simulink model "complete_model"  (R2023b)
settings: Solver=ode5  StartTime=0.0  StopTime=1000  RelTol=1e-3
values from neighbouring files (symbols this model uses):
  a = 6851.22197053    [IGRF13_2020.mat]    (also in complete_model.m; complete_model_main.m; loop_model.m; orbit_plot_report.m)
  alpha1 = 0.4    [IGRF13_2020.mat]    (also in complete_model.m = 0.05; complete_model_main.m; loop_model.m)
  alpha2 = 0.1    [IGRF13_2020.mat]    (also in complete_model.m = 0.15; complete_model_main.m; loop_model.m)
  alpha3 = 0.5    [IGRF13_2020.mat]    (also in complete_model.m = 0.8; complete_model_main.m; loop_model.m)
  e = 0.00183012221618    [IGRF13_2020.mat]    (also in complete_model.m; complete_model_main.m; loop_model.m; orbit_plot_report.m)
  FOV_earth = 0.575958653158    [IGRF13_2020.mat]    (also in complete_model.m = deg2rad(33); complete_model_main.m = deg2rad(33); loop_model.m = deg2rad(33))
  FOV_sun = deg2rad(85)    [complete_model_main.m]
  freq_earth = 30    [IGRF13_2020.mat]    (also in complete_model.m; complete_model_main.m = 5; loop_model.m)
  freq_mag = 30    [IGRF13_2020.mat]    (also in complete_model.m; complete_model_main.m = 5; loop_model.m)
  freq_sun = 30    [IGRF13_2020.mat]    (also in complete_model.m; complete_model_main.m = 5; loop_model.m)
  H0 = 2.98059244128e-05    [IGRF13_2020.mat]    (also in complete_model.m = sqrt(g01^2+g11^2+h11^2)*1e-9; complete_model_main.m = sqrt(g01^2+g11^2+h11^2)*1e-9; loop_model.m = sqrt(g01^2+g11^2+h11^2)*1e-9)
  I = diag([I1 I2 I3])    [complete_model_main.m]
  Iinv = I\eye(3)    [complete_model_main.m]
  incl = 0.200712863979    [IGRF13_2020.mat]    (also in complete_model.m = deg2rad(11.5); complete_model_main.m = deg2rad(11.5); loop_model.m = deg2rad(11.5))
  jb = [0.01 0.05 0.01]    [IGRF13_2020.mat]    (also in complete_model.m = [0.01; 0.05; 0.01]; complete_model_main.m = [0.01; 0.05; 0.01]; loop_model.m = [0.01; 0.05; 0.01])
  k_gain = 0.0363323388759    [IGRF13_2020.mat]    (also in complete_model.m = (4*pi/T) * (1 + sin(chsi)) * I1_retr; complete_model_main.m = (4*pi/T) * (1 + sin(chsi)) * min([I1, I2, I3]); loop_model.m = (4*pi/T) * (1 + sin(chsi)) * I1_retr)
  max_dip = 15    [IGRF13_2020.mat]    (also in complete_model.m; complete_model_main.m = 150; loop_model.m)
  mu = 398600.433    [IGRF13_2020.mat]    (also in complete_model.m = astroConstants(13); complete_model_main.m = astroConstants(13); loop_model.m = astroConstants(13); orbit_plot_report.m = astroConstants(13))
  n = 0.00111331183439    [IGRF13_2020.mat]    (also in complete_model.m = sqrt(mu/a^3); complete_model_main.m = sqrt(mu/a^3); loop_model.m = sqrt(mu/a^3); orbit_plot_report.m = sqrt(mu/a^3))
  omega0 = [0.06 0.06 0.06]    [IGRF13_2020.mat]    (also in complete_model.m = -0.06 + 0.12 * rand(3,1); complete_model_main.m = [0.01; 0.01; 0.01]*6; init_cond.mat = [-0.0472016675783 0.0554277697026 -0.0594438931039]; loop_model.m = 0.06 * ones(3,1))
  omegaE = 7.27220521664e-05    [IGRF13_2020.mat]    (also in complete_model.m = deg2rad(15)/3600; complete_model_main.m = deg2rad(15)/3600; loop_model.m = deg2rad(15)/3600)
  rs = [-16878165.0145 -134206589.72 -58177126.6728]    [IGRF13_2020.mat]    (also in complete_model.m = -rr; complete_model_main.m = -rr; loop_model.m = -rr; orbit_plot_report.m = -rr)
  Rt = 6371.01    [IGRF13_2020.mat]    (also in Terra_3D.m = 6378.1363; complete_model.m = astroConstants(23); complete_model_main.m = astroConstants(23); loop_model.m = astroConstants(23))
  s0 = [6.01405730572 3.04970514452 5.02831048374]    [IGRF13_2020.mat]    (also in buonnatale.mat = [2.59731710564 0.831637671153 -2.52872821404]; complete_model.m = 2*pi*rand(3,1); complete_model_main.m = -pi + 2 * pi * rand(3,1); init_cond.mat = [4.86890604626 5.13526758752 5.45816980916])
  tol = 0.2    [IGRF13_2020.mat]    (also in complete_model.m; complete_model_main.m; loop_model.m)
undefined symbols (not defined in the file or in its folder): magnitude
libraries: matrix_library x8, vrlib x8, simulink x7, sharedutil x2, dspmathops x2, dspfactors x1, cstblocks x1
(part 2 of 2)

== system complete_model/Kinematics/Kinematics 313/s_312 - A/R2 ==
  x : Inport
  Constant : Constant  Value=[0; 1; 0]
  Constant1 : Constant  Value=0
  Cos : Trigonometry  Operator=cos
  Gain : Gain  Gain=-1
  Matrix Concatenate : Concatenate  NumInputs=3  Mode=Multidimensional array  ConcatenateDimension=2
  Sin : Trigonometry
  Vector Concatenate : Concatenate  NumInputs=3
  Vector Concatenate1 : Concatenate  NumInputs=3
  R2 : Outport
  wires:
  Vector Concatenate/1 -> Matrix Concatenate/1
  x/1 -> Sin/1, Cos/1
  Matrix Concatenate/1 -> R2/1
  Constant/1 -> Matrix Concatenate/2
  Vector Concatenate1/1 -> Matrix Concatenate/3
  Constant1/1 -> Vector Concatenate/2, Vector Concatenate1/2
  Cos/1 -> Vector Concatenate1/3, Vector Concatenate/1
  Sin/1 -> Gain/1, Vector Concatenate/3
  Gain/1 -> Vector Concatenate1/1

== system complete_model/Kinematics/Kinematics 313/s_312 - A/R3 ==
  x : Inport
  Constant : Constant  Value=[0; 0; 1]
  Constant1 : Constant  Value=0
  Cos : Trigonometry  Operator=cos
  Gain : Gain  Gain=-1
  Matrix Concatenate : Concatenate  NumInputs=3  Mode=Multidimensional array  ConcatenateDimension=2
  Sin : Trigonometry
  Vector Concatenate : Concatenate  NumInputs=3
  Vector Concatenate1 : Concatenate  NumInputs=3
  R3 : Outport
  wires:
  Vector Concatenate/1 -> Matrix Concatenate/1
  Sin/1 -> Vector Concatenate1/1, Gain/1
  Cos/1 -> Vector Concatenate1/2, Vector Concatenate/1
  Constant/1 -> Matrix Concatenate/3
  Gain/1 -> Vector Concatenate/2
  Vector Concatenate1/1 -> Matrix Concatenate/2
  x/1 -> Sin/1, Cos/1
  Constant1/1 -> Vector Concatenate/3, Vector Concatenate1/3
  Matrix Concatenate/1 -> R3/1

== system complete_model/Kinematics/Kinematics 313/s_313 - A/R1 ==
  x : Inport
  Constant : Constant  Value=[1; 0; 0]
  Constant1 : Constant  Value=0
  Cos : Trigonometry  Operator=cos
  Gain : Gain  Gain=-1
  Matrix Concatenate : Concatenate  NumInputs=3  Mode=Multidimensional array  ConcatenateDimension=2
  Sin : Trigonometry
  Vector Concatenate : Concatenate  NumInputs=3
  Vector Concatenate1 : Concatenate  NumInputs=3
  R1 : Outport
  wires:
  Sin/1 -> Gain/1, Vector Concatenate/2
  Gain/1 -> Vector Concatenate1/3
  Cos/1 -> Vector Concatenate1/2, Vector Concatenate/3
  Constant1/1 -> Vector Concatenate1/1, Vector Concatenate/1
  Vector Concatenate/1 -> Matrix Concatenate/3
  Constant/1 -> Matrix Concatenate/1
  Vector Concatenate1/1 -> Matrix Concatenate/2
  x/1 -> Sin/1, Cos/1
  Matrix Concatenate/1 -> R1/1

== system complete_model/Kinematics/Kinematics 313/s_313 - A/R3_1 ==
  x : Inport
  Constant : Constant  Value=[0; 0; 1]
  Constant1 : Constant  Value=0
  Cos : Trigonometry  Operator=cos
  Gain : Gain  Gain=-1
  Matrix Concatenate : Concatenate  NumInputs=3  Mode=Multidimensional array  ConcatenateDimension=2
  Sin : Trigonometry
  Vector Concatenate : Concatenate  NumInputs=3
  Vector Concatenate1 : Concatenate  NumInputs=3
  R3 : Outport
  wires:
  Matrix Concatenate/1 -> R3/1
  Constant1/1 -> Vector Concatenate1/3, Vector Concatenate/3
  x/1 -> Cos/1, Sin/1
  Vector Concatenate1/1 -> Matrix Concatenate/2
  Gain/1 -> Vector Concatenate/2
  Constant/1 -> Matrix Concatenate/3
  Cos/1 -> Vector Concatenate/1, Vector Concatenate1/2
  Sin/1 -> Gain/1, Vector Concatenate1/1
  Vector Concatenate/1 -> Matrix Concatenate/1

== system complete_model/Kinematics/Kinematics 313/s_313 - A/R3_2 ==
  x : Inport
  Constant : Constant  Value=[0; 0; 1]
  Constant1 : Constant  Value=0
  Cos : Trigonometry  Operator=cos
  Gain : Gain  Gain=-1
  Matrix Concatenate : Concatenate  NumInputs=3  Mode=Multidimensional array  ConcatenateDimension=2
  Sin : Trigonometry
  Vector Concatenate : Concatenate  NumInputs=3
  Vector Concatenate1 : Concatenate  NumInputs=3
  R3 : Outport
  wires:
  Vector Concatenate/1 -> Matrix Concatenate/1
  Sin/1 -> Vector Concatenate1/1, Gain/1
  Cos/1 -> Vector Concatenate1/2, Vector Concatenate/1
  Constant/1 -> Matrix Concatenate/3
  Gain/1 -> Vector Concatenate/2
  Vector Concatenate1/1 -> Matrix Concatenate/2
  x/1 -> Sin/1, Cos/1
  Constant1/1 -> Vector Concatenate/3, Vector Concatenate1/3
  Matrix Concatenate/1 -> R3/1
